simulink model "BuildingModelWithSolarLoad"  (R2024a)
settings: Solver=ode1be  StartTime=0.0  StopTime=522000  FixedStep=3600  MaxStep=3600  RelTol=1e-3  AbsTol=1e-3
PreLoadFcn:
  | % WallModelParams
libraries: fl_lib x12, nesl_utility x6
CloseFcn:
  | % clear flow out roomHeight wall win
settings Model: Creator=vikrants  LastModifiedBy=vikrants
settings SolverCC: AutoScaleAbsTol=off  AlgebraicLoopSolver=TrustRegion  MaxZcPerStep=1
settings DebuggingCC: UnconnectedInputMsg=warning  UnconnectedOutputMsg=warning  UnconnectedLineMsg=warning  SymbolicDimsDataTypeCodeGenerationDiagnostic=none
settings ModelReferenceCC: EnableRefExpFcnMdlSchedulingChecks=on
settings SFSimCC: CustomCodeUndefinedFunction=UseInterfaceOnly
settings RTWCC: GPUComputeCapability=3.5  DLArmComputeVersion=19.05
settings SimscapeCC: SimscapeLogType=all  SimscapeLogSimulationStatistics=on  SimscapeLogLimitData=off  SimscapeLogDataHistory=10000  SimscapeCompileComponentReuse=on  SimscapeMultithreadedCompilation=off

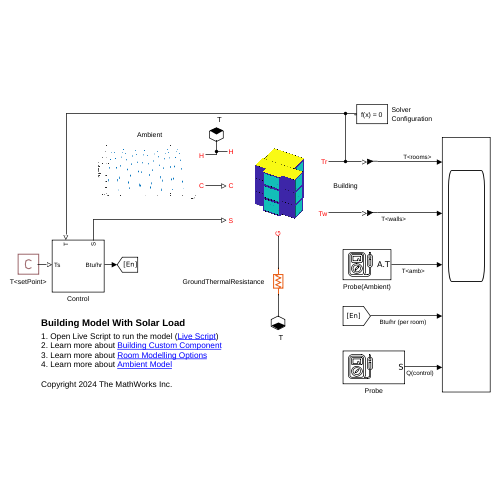
[thumbnail: Simulink's stored preview of the top-level diagram]
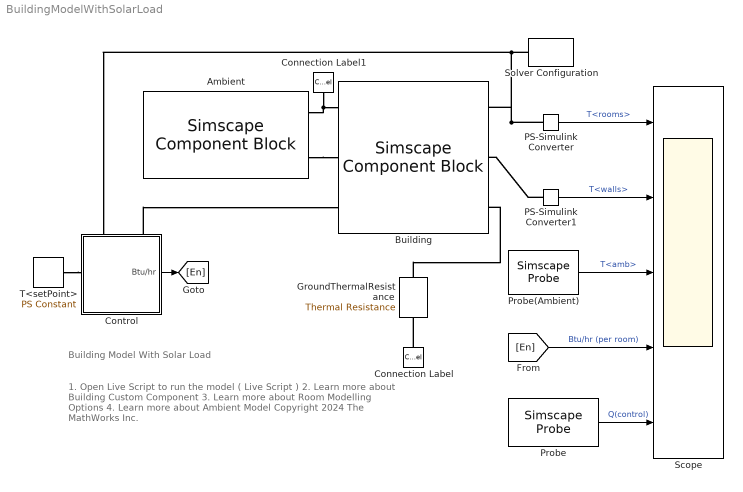
== system BuildingModelWithSolarLoad ==
  note: 1. Open Live Script to run the model ( Live Script )
      | 2. Learn more about Building Custom Component
      | 3. Learn more about Room Modelling Options
      | 4. Learn more about Ambient Model
      |
      | Copyright 2024 The MathWorks Inc.
  note: Building Model With Solar Load
  Ambient : SimscapeComponentBlock  SourceFile=EnvModel  ComponentPath=EnvModel  ComponentVariants="[\"EnvModel\"]"  ComponentVariantNames="[\"EnvModel\"]"  ClassName=EnvModel  SchemaVersion=1  listOfDays="[122  123  124  125  126  127  128] % Parameterized on :13-Nov-2024 08:59:39"  sunrise="[19381.846      19356.8068      19332.5383       19309.053      19286.3628      19264.4789      19243.4119] % Parameterized on :13-Nov-2024 08:59:39 s"  sunset="[67018.154      67043.1932      67067.4617       67090.947      67113.6372      67135.5211      67156.5881] % Parameterized on :13-Nov-2024 08:59:39 s"  startTime=3600 % Parameterized on :13-Nov-2024 08:59:39 s  avgDayTvec="[303  303  303  303  303  303  303] % Parameterized on :13-Nov-2024 08:59:39 K"  pcDayTvar=1 % Parameterized on :13-Nov-2024 08:59:39  avgNightTvec="[299  299  299  299  299  299  299] % Parameterized on :13-Nov-2024 08:59:39 K"  pcNightTvar=1 % Parameterized on :13-Nov-2024 08:59:39  cloudData=cloudCoverOptions.daily  cloudCoverVal="[0  0  0  0  0  0  0] % Parameterized on :13-Nov-2024 08:59:39"
      settings: CopyFcn=simscape.engine.sli.internal.componentblockcallback(gcbh,'COPY')  PreCopyFcn=simscape.engine.sli.internal.componentblockcallback(gcbh,'PRECOPY')  PreDeleteFcn=simscape.engine.sli.internal.componentblockcallback(gcbh,'PREDELETE')  InternalSimscapePortConfiguration="{\"Bottom\":[],\"Left\":[],\"Right\":[{\"id\":\"A\",\"label\":\"H\",\"type\":\"foundation.thermal.thermal\"},{\"id\":\"cloud\",\"label\":\"C\",\"type\":\"output\"}],\"Top\":[]}"
      mask Type: EnvModel
  Building : SimscapeComponentBlock  SourceFile=BuildingModel  ComponentPath=BuildingModel  ComponentVariants="[\"BuildingModel\"]"  ComponentVariantNames="[\"BuildingModel\"]"  ClassName=BuildingModel  SchemaVersion=1  nApts=3 % Parameterized on :13-Nov-2024 08:59:39  nRooms=4 % Parameterized on :13-Nov-2024 08:59:39  roomVolMat=[22.6534772736 39.6435852288 13.59208636416 9.9108963072;22.6534772736 39.6435852288 13.59208636416 9.9108963072;22.6534772736 39.6435852288 13.59208636416 9.9108963072] % Parameterized on :13-Nov-2024 08:59:39 m^3  roomConnMat=[1 1 1 2 1.9235928;1 1 1 3 7.1789544;1 1 1 4 6.2816232;1 2 1 3 0.48121824;1 2 1 4 0.9614916;2 1 2 2 1.9235928;2 1 2 3 7.1789544;2 1 2 4 6.2816232;2 2 2 3 0.48121824;2 2 2 4 0.9614916;3 1 3 2 1.9235928;3 1 3 3 7.1789544;3 1 3 4 6.2816232;3 2 3 3 0.48121824;3 2 3 4 0.9614916;1 1 2 1 7.4322432;1 2 2 2 13.0064256;1 3 2 3 4.45934592;1 4 2 4 3.2516064;2 1 3 1 7.4322432;2 2 3 2 13.0064256;2 3 3 3 4.45934592;2 4 3 4 3.2516064] % Parameterized on :13-Nov-2024 08:59:39  roomEnvConnMat=[1 1 1 2.22966 5.20254 0;1 1 2 2.536809318 0 0;1 1 4 3.094691833 0 0;1 2 2 9.2903 0 0;1 2 3 3.90192 9.10448 0;1 2 4 4.64515 4.64515 0;1 3 1 5.5742 0 0;1 3 3 1.165788188 0 0;1 3 4 2.22966 5.20254 0;1 4 1 4.6452 0 0;1 4 2 4.55224 1.95096 0;1 4 3 0.8698137 0 0;2 1 1 2.22966 5.20254 0;2 1 2 2.536809318 0 0;2 1 4 3.094691833 0 0;2 2 2 9.2903 0 0;2 2 3 3.90192 9.10448 0;2 2 4 4.64515 4.64515 0;2 3 1 5.5742 0 0;2 3 3 1.165788188 0 0;2 3 4 2.22966 5.20254 0;2 4 1 4.6452 0 0;2 4 2 4.55224 1.95096 0;2 4 3 0.8698137 0 0;3 1 1 2.22966 5.20254 0;3 1 2 2.536809318 0 0;3 1 4 3.094691833 0 0;3 2 2 9.2903 0 0;3 2 3 3.90192 9.10448 0;3 2 4 4.64515 4.64515 0;3 3 1 5.5742 0 0;3 3 3 1.165788188 0 0;3 3 4 2.22966 5.20254 0;3 4 1 4.6452 0 0;3 4 2 4.55224 1.95096 0;3 4 3 0.8698137 0 0] % Parameterized on :13-Nov-2024 08:59:39  roomEnvSolarRad=[0 0 0 0 0 0 0 0 0 0 0 0 508.7493 695.7679 740.5149 646.0261 443.1172 175.983 0 0 0 0 0 0 0 0 0 0 0 0 0 0 0 0 0 0 506.6863 693.3518 738.2975 644.5609 442.8175 177.0738 0 0 0 0 0 0 0 0 0 0 0 0 0 0 0 0 0 0 504.6328 690.9373 736.0614 643.0554 442.4581 178.0902 0 0 0 0 0 0 0 0 0 0 0 0 0 0 0 0 0 0 502.5917 688.5273 733.8098 641.5122 442.0409 179.033 0 0 0 0 0 0 0 0 0 0 0 0 0 0 0 0 0 0 500.5659 686.125 731.5459 639.9341 441.5678 179.9031 0 0 0 0 0 0 0 0 0 0 0 0 0 0 0 0 0 0 498.5584 683.7335 729.2727 638.3238 441.0408 180.7014 0 0 0 0 0 0 0;0 0 0 0 0 0 0 0 0 0 0 0 0 0 0 0 0 0 0 0 0 0 0 0 0 0 0 0 0 0 0 0 0 0 0 0 0 0 0 0 0 0 0 0 0 0 0 0 0 0 0 0 0 0 0 0 0 0 0 0 0 0 0 0 0 0 0 0 0 0 0 0 0 0 0 0 0 0 0 0 0 0 0 0 0 0 0 0 0 0 0 0 0 0 0 0 0 0 0 0 0 0 0 0 0 0 0 0 0 0 0 0 0 0 0 0 0 0 0 0 0 0 0 0 0 0 0 0 0 0 0 0 0 0 0 0 0 0 0 0 0 0 0 0 0;0 0 0 0 0 0 8.760353 103.49157 342.38462 691.35726 1034.3368 1231.5064 0 0 0 0 0 0 0 0 0 0 0 0 0 0 0 0 0 0 7.2840779 100.4301 337.93248 686.02689 1029.0281 1226.9589 1091.7999 0 0 0 0 0 0 0 0 0 0 0 0 0 0 0 0 0 5.8286813 97.427164 333.55914 680.76079 1023.7247 1222.29 1088.064 0 0 0 0 0 0 0 0 0 0 0 0 0 0 0 0 0 4.3944434 94.483934 329.26741 675.5639 1018.4336 1217.5127 1084.1895 0 0 0 0 0 0 0 0 0 0 0 0 0 0 0 0 0 2.98164 91.601534 325.05996 670.44102 1013.1618 1212.6398 1080.1838 0 0 0 0 0 0 0 0 0 0 0 0 0 0 0 0 0 1.5905448 88.78103 320.93937 665.39687 1007.9163 1207.6841 1076.055 0 0 0 0 0 0 0 0 0 0 0 0;0 0 0 0 0 0 0 0 0 0 0 0 0 0 0 0 0 0 0 0 0 0 0 0 0 0 0 0 0 0 0 0 0 0 0 0 0 0 0 0 0 0 0 0 0 0 0 0 0 0 0 0 0 0 0 0 0 0 0 0 0 0 0 0 0 0 0 0 0 0 0 0 0 0 0 0 0 0 0 0 0 0 0 0 0 0 0 0 0 0 0 0 0 0 0 0 0 0 0 0 0 0 0 0 0 0 0 0 0 0 0 0 0 0 0 0 0 0 0 0 0 0 0 0 0 0 0 0 0 0 0 0 0 0 0 0 0 0 0 0 0 0 0 0 0;0 0 0 0 0 0 0 0 0 0 0 0 0 0 0 0 0 0 0 0 0 0 0 0 0 0 0 0 0 0 0 0 0 0 0 0 0 0 0 0 0 0 0 0 0 0 0 0 0 0 0 0 0 0 0 0 0 0 0 0 0 0 0 0 0 0 0 0 0 0 0 0 0 0 0 0 0 0 0 0 0 0 0 0 0 0 0 0 0 0 0 0 0 0 0 0 0 0 0 0 0 0 0 0 0 0 0 0 0 0 0 0 0 0 0 0 0 0 0 0 0 0 0 0 0 0 0 0 0 0 0 0 0 0 0 0 0 0 0 0 0 0 0 0 0;0 0 0 0 0 0 8.760353 103.49157 342.38462 691.35726 1034.3368 1231.5064 0 0 0 0 0 0 0 0 0 0 0 0 0 0 0 0 0 0 7.2840779 100.4301 337.93248 686.02689 1029.0281 1226.9589 1091.7999 0 0 0 0 0 0 0 0 0 0 0 0 0 0 0 0 0 5.8286813 97.427164 333.55914 680.76079 1023.7247 1222.29 1088.064 0 0 0 0 0 0 0 0 0 0 0 0 0 0 0 0 0 4.3944434 94.483934 329.26741 675.5639 1018.4336 1217.5127 1084.1895 0 0 0 0 0 0 0 0 0 0 0 0 0 0 0 0 0 2.98164 91.601534 325.05996 670.44102 1013.1618 1212.6398 1080.1838 0 0 0 0 0 0 0 0 0 0 0 0 0 0 0 0 0 1.5905448 88.78103 320.93937 665.39687 1007.9163 1207.6841 1076.055 0 0 0 0 0 0 0 0 0 0 0 0;0 0 0 0 0 0 0 0 0 0 0 0 508.7493 695.7679 740.5149 646.0261 443.1172 175.983 0 0 0 0 0 0 0 0 0 0 0 0 0 0 0 0 0 0 506.6863 693.3518 738.2975 644.5609 442.8175 177.0738 0 0 0 0 0 0 0 0 0 0 0 0 0 0 0 0 0 0 504.6328 690.9373 736.0614 643.0554 442.4581 178.0902 0 0 0 0 0 0 0 0 0 0 0 0 0 0 0 0 0 0 502.5917 688.5273 733.8098 641.5122 442.0409 179.033 0 0 0 0 0 0 0 0 0 0 0 0 0 0 0 0 0 0 500.5659 686.125 731.5459 639.9341 441.5678 179.9031 0 0 0 0 0 0 0 0 0 0 0 0 0 0 0 0 0 0 498.5584 683.7335 729.2727 638.3238 441.0408 180.7014 0 0 0 0 0 0 0;0 0 0 0 0 0 0 0 0 0 0 0 0 0 0 0 0 0 0 0 0 0 0 0 0 0 0 0 0 0 0 0 0 0 0 0 0 0 0 0 0 0 0 0 0 0 0 0 0 0 0 0 0 0 0 0 0 0 0 0 0 0 0 0 0 0 0 0 0 0 0 0 0 0 0 0 0 0 0 0 0 0 0 0 0 0 0 0 0 0 0 0 0 0 0 0 0 0 0 0 0 0 0 0 0 0 0 0 0 0 0 0 0 0 0 0 0 0 0 0 0 0 0 0 0 0 0 0 0 0 0 0 0 0 0 0 0 0 0 0 0 0 0 0 0;0 0 0 0 0 0 8.760353 103.49157 342.38462 691.35726 1034.3368 1231.5064 0 0 0 0 0 0 0 0 0 0 0 0 0 0 0 0 0 0 7.2840779 100.4301 337.93248 686.02689 1029.0281 1226.9589 1091.7999 0 0 0 0 0 0 0 0 0 0 0 0 0 0 0 0 0 5.8286813 97.427164 333.55914 680.76079 1023.7247 1222.29 1088.064 0 0 0 0 0 0 0 0 0 0 0 0 0 0 0 0 0 4.3944434 94.483934 329.26741 675.5639 1018.4336 1217.5127 1084.1895 0 0 0 0 0 0 0 0 0 0 0 0 0 0 0 0 0 2.98164 91.601534 325.05996 670.44102 1013.1618 1212.6398 1080.1838 0 0 0 0 0 0 0 0 0 0 0 0 0 0 0 0 0 1.5905448 88.78103 320.93937 ...(+11544 chars)] % Parameterized on :13-Nov-2024 08:59:39  floorGroundConn=[1 1 7.4322432;1 2 13.0064256;1 3 4.45934592;1 4 3.2516064] % Parameterized on :13-Nov-2024 08:59:39  roomModelOption=roomPhysicsOptions.requirements  roomRadiatorArea=ones(5, 8) m^2  roomUFPipingArea=ones(5, 8) m^2  roofEnvConnMat=[3 1 7.4322432;3 2 13.0064256;3 3 4.45934592;3 4 3.2516064] % Parameterized on :13-Nov-2024 08:59:39  roofEnvSolarRad=[0 0 0 0 0 0 59.37688 284.0187 558.4148 731.6277 703.3205 481.3691 548.3154 730.7268 705.3155 494.6307 218.2659 27.22395 0 0 0 0 0 0 0 0 0 0 0 0 59.62248 284.8127 560.2036 735.0546 709.0017 490.7252 555.3351 735.4838 708.7842 497.1489 219.8792 27.78296 0 0 0 0 0 0 0 0 0 0 0 0 59.88223 285.6142 561.9659 738.4099 714.5914 500.0937 562.4302 740.1887 712.1618 499.5757 221.4311 28.32576 0 0 0 0 0 0 0 0 0 0 0 0 60.15639 286.4239 563.703 741.6939 720.0859 509.4443 569.5843 744.8379 715.4469 501.9099 222.9203 28.85136 0 0 0 0 0 0 0 0 0 0 0 0 60.44522 287.2427 565.4158 744.9067 725.4816 518.7498 576.781 749.4277 718.6383 504.1509 224.3458 29.3588 0 0 0 0 0 0 0 0 0 0 0 0 60.74897 288.0714 567.1056 748.0487 730.7754 527.9854 584.0035 753.9547 721.7348 506.2978 225.7066 29.84717 0 0 0 0 0 0 0;0 0 0 0 0 0 59.37688 284.0187 558.4148 731.6277 703.3205 481.3691 548.3154 730.7268 705.3155 494.6307 218.2659 27.22395 0 0 0 0 0 0 0 0 0 0 0 0 59.62248 284.8127 560.2036 735.0546 709.0017 490.7252 555.3351 735.4838 708.7842 497.1489 219.8792 27.78296 0 0 0 0 0 0 0 0 0 0 0 0 59.88223 285.6142 561.9659 738.4099 714.5914 500.0937 562.4302 740.1887 712.1618 499.5757 221.4311 28.32576 0 0 0 0 0 0 0 0 0 0 0 0 60.15639 286.4239 563.703 741.6939 720.0859 509.4443 569.5843 744.8379 715.4469 501.9099 222.9203 28.85136 0 0 0 0 0 0 0 0 0 0 0 0 60.44522 287.2427 565.4158 744.9067 725.4816 518.7498 576.781 749.4277 718.6383 504.1509 224.3458 29.3588 0 0 0 0 0 0 0 0 0 0 0 0 60.74897 288.0714 567.1056 748.0487 730.7754 527.9854 584.0035 753.9547 721.7348 506.2978 225.7066 29.84717 0 0 0 0 0 0 0;0 0 0 0 0 0 59.37688 284.0187 558.4148 731.6277 703.3205 481.3691 548.3154 730.7268 705.3155 494.6307 218.2659 27.22395 0 0 0 0 0 0 0 0 0 0 0 0 59.62248 284.8127 560.2036 735.0546 709.0017 490.7252 555.3351 735.4838 708.7842 497.1489 219.8792 27.78296 0 0 0 0 0 0 0 0 0 0 0 0 59.88223 285.6142 561.9659 738.4099 714.5914 500.0937 562.4302 740.1887 712.1618 499.5757 221.4311 28.32576 0 0 0 0 0 0 0 0 0 0 0 0 60.15639 286.4239 563.703 741.6939 720.0859 509.4443 569.5843 744.8379 715.4469 501.9099 222.9203 28.85136 0 0 0 0 0 0 0 0 0 0 0 0 60.44522 287.2427 565.4158 744.9067 725.4816 518.7498 576.781 749.4277 718.6383 504.1509 224.3458 29.3588 0 0 0 0 0 0 0 0 0 0 0 0 60.74897 288.0714 567.1056 748.0487 730.7754 527.9854 584.0035 753.9547 721.7348 506.2978 225.7066 29.84717 0 0 0 0 0 0 0;0 0 0 0 0 0 59.37688 284.0187 558.4148 731.6277 703.3205 481.3691 548.3154 730.7268 705.3155 494.6307 218.2659 27.22395 0 0 0 0 0 0 0 0 0 0 0 0 59.62248 284.8127 560.2036 735.0546 709.0017 490.7252 555.3351 735.4838 708.7842 497.1489 219.8792 27.78296 0 0 0 0 0 0 0 0 0 0 0 0 59.88223 285.6142 561.9659 738.4099 714.5914 500.0937 562.4302 740.1887 712.1618 499.5757 221.4311 28.32576 0 0 0 0 0 0 0 0 0 0 0 0 60.15639 286.4239 563.703 741.6939 720.0859 509.4443 569.5843 744.8379 715.4469 501.9099 222.9203 28.85136 0 0 0 0 0 0 0 0 0 0 0 0 60.44522 287.2427 565.4158 744.9067 725.4816 518.7498 576.781 749.4277 718.6383 504.1509 224.3458 29.3588 0 0 0 0 0 0 0 0 0 0 0 0 60.74897 288.0714 567.1056 748.0487 730.7754 527.9854 584.0035 753.9547 721.7348 506.2978 225.7066 29.84717 0 0 0 0 0 0 0] % Parameterized on :13-Nov-2024 08:59:39  radiatorPipeGap=1e-2 m  radiatorPipeHydrDia=5e-3 m  radiatorPipeArea=2e-5 m^2  UFPipeGap=1e-1 m  UFPipeHydrDia=5e-3 m  UFPipeArea=2e-5 m^2  wallAbsorptivity=.6  wallThickness=0.3 m  wallMaterialDen=2400 kg/m^3  wallMaterialCp=1500 J/(K*kg)  wallThermalK=2.25 W/(K*m)  winAbsorptivity=.4  winTransmissivity=.2  winThickness=.01 m  winMaterialDen=4000 kg/m^3  winMaterialCp=840 J/(K*kg)  winThermalK=1 W/(K*m)  heatTransferPipeRoughness=1e-06 m  extToWallHTC=5 W/(K*m^2)  intToRoomHTC=5 W/(K*m^2)  iniTemperature=299 % Parameterized on :13-Nov-2024 08:59:39 K  airDensity=1.28 kg/m^3  airCp=700 J/(K*kg)  minArea=1e-10 m^2
      settings: CopyFcn=simscape.engine.sli.internal.componentblockcallback(gcbh,'COPY')  PreCopyFcn=simscape.engine.sli.internal.componentblockcallback(gcbh,'PRECOPY')  PreDeleteFcn=simscape.engine.sli.internal.componentblockcallback(gcbh,'PREDELETE')  InternalSimscapePortConfiguration="{\"Bottom\":[{\"id\":\"G\",\"label\":\"G\",\"type\":\"foundation.thermal.thermal\"}],\"Left\":[{\"id\":\"H\",\"label\":\"H\",\"type\":\"foundation.thermal.thermal\"},{\"id\":\"C\",\"label\":\"C\",\"type\":\"input\"},{\"id\":\"S\",\"label\":\"S\",\"type\":\"input\"}],\"Right\":[{\"id\":\"roomTemp\",\"label\":\"Tr\",\"type\":\"output\"},{\"id\":\"wallTemp\",\"label\":\"Tw\",\"type\":\"output\"}],\"Top\":[]}"
      mask Type: BuildingModel
  Connection Label : ConnectionLabel  Label=T
  Connection Label1 : ConnectionLabel  Label=T
  Control : Subsystem
      settings: PortSchema="{\"entries\":[{\"content\":{\"sides\":[{\"content\":{\"connectorIds\":[\"Out1\"]},\"type\":\"ConnectorPlacement.EquallySpacedRectSide\",\"uuid\":\"bf0d3f6c-4199-48ed-9d1b-942d678a196d\"},{\"content\":{\"connectorIds\":[\"RConn1\"],\"side\":\"RIGHT\"},\"type\":\"ConnectorPlacement.EquallySpacedRectSide\",\"uuid\":\"048b5b2b-ccfc-4083-80b1-51c1896923e2\"},{\"content\":{\"side\":\"TOP\"},\"type\":\"ConnectorPlacement.EquallySpacedRectSide\",\"uuid\":\"550f74ea-2758-4466-8134-2f10276d8ab6\"},{\"content\":{\"connectorIds\":[\"RConn2\",\"RConn3\"],\"side\":\"BOTTOM\"},\"type\":\"ConnectorPlacement.EquallySpacedRectSide\",\"uuid\":\"b8e21315-4710-4fb3-a2ab-c08e79356caa\"}]},\"type\":\"ConnectorPlacement.EquallySpacedConnector\",\"uuid\":\"91aadc23-894a-4dd0-ab72-650090e5f490\"}],\"packageUris\":[\"http://schema.mathworks.com/mf0/Connector/R2020b\"],\"version\":\"1.0\"}"
  GroundThermalResistance : fl_lib/Thermal/Thermal Elements/Thermal Resistance  resistance=100 % Parameterized on :13-Nov-2024 08:59:39 K/W  T_specify=off  T_priority=None  T=0 K  T_nominal_specify=off  T_nominal_value=1  T_nominal_unit=K  Q_specify=off  Q_priority=None  Q=0 W  Q_nominal_specify=off  Q_nominal_value=1  Q_nominal_unit=W
  PS-Simulink Converter : nesl_utility/PS-Simulink Converter  PhysicalDomain=network_engine_domain  SubClassName=ps_output  LeftPortType=input  RightPortType=output  PseudoPeriodic=off  Frequencies=[]  VectorFormat=inherit  Unit=inherit  AffineConversion=off
  PS-Simulink Converter1 : nesl_utility/PS-Simulink Converter  PhysicalDomain=network_engine_domain  SubClassName=ps_output  LeftPortType=input  RightPortType=output  PseudoPeriodic=off  Frequencies=[]  VectorFormat=inherit  Unit=inherit  AffineConversion=off
  Probe : SimscapeProbe  BoundBlock=49  Variables={S}
  Probe(Ambient) : SimscapeProbe  BoundBlock=267  Variables={A.T}
  Scope : Scope  NumInputPorts=5
  Solver Configuration : nesl_utility/Solver Configuration  PhysicalDomain=network_engine_domain  SubClassName=solver  LeftPortType=input  RightPortType=generic  Tones=[]  Harmonics=[]  SimulateNoise=off  Profile=off  UseLocalSampling=off  EnableSwitchedLinearOptims=on  FrequencyDomain=off  UseCCode=off  RelTol=0.001  AbsTol=1e-06  MinStep=1e-09  ToWorkspace=off  RevertToSquareIcSolve=off  NumHomotopyIterations=100  PhasorMode=off  PhasorModeNumHarmonics=1  ConsistencySolver=NEWTON_XTOL_AFTER_FTOL  IndexReductionMethod=DerivativeReplacement  DoDC=off  ResidualTolerance=1e-09  ConsistencyTolSource=GLOBAL  ConsistencyAbsTol=0.001  ConsistencyRelTol=0.001  ConsistencyTolFactor=0.001  UseLocalSolver=off  LocalSolverChoice=NE_BACKWARD_EULER_ADVANCER  ResolveIndetEquations=on  FunctionEvalNumThread=1  LocalSolverSampleTime=3600  DoFixedCost=off  MaxNonlinIter=3  MaxModeIter=2  ComputeImpulses=off  ImpulseIterations=2  LinearAlgebra=auto  LinearAlgebraNumThread=0  EquationFormulation=NE_TIME_EF  DelaysMemoryBudget=1024  AutomaticFiltering=on  FilteringTimeConstant=0.001  PartitionStorageMethod=AS_NEEDED  PartitionMemoryBudget=1024  PartitionMethod=ROBUST  MultibodyUseLocalSolver=off  MultibodyLocalSolverChoice=ODE1  MultibodyLocalSolverSampleTime=0.001
  T<setPoint> : fl_lib/Physical Signals/Sources/PS Constant  constant=293 % Parameterized on :13-Nov-2024 08:59:39 K
  wires:
  Probe(Ambient)/1 -> Scope/3  "T<amb>"
  PS-Simulink Converter/1 -> Scope/1  "T<rooms>"
  PS-Simulink Converter1/1 -> Scope/2  "T<walls>"
  Control/1(Btu/hr) -> [En]
  [En] -> Scope/4  "Btu/hr (per room)"
  Probe/1 -> Scope/5  "Q(control)"
  connections:
  PS-Simulink Converter1/LConn1 -- Building/RConn2
  Ambient/RConn1 -- Connection Label1/LConn1 -- Building/LConn1
  PS-Simulink Converter/LConn1 -- Solver Configuration/RConn1 -- Control/RConn3 -- Building/RConn1
  Control/RConn2 -- Building/LConn3
  T<setPoint>/RConn1 -- Control/RConn1
  Ambient/RConn2 -- Building/LConn2
  Connection Label/LConn1 -- GroundThermalResistance/RConn1
  GroundThermalResistance/LConn1 -- Building/RConn3

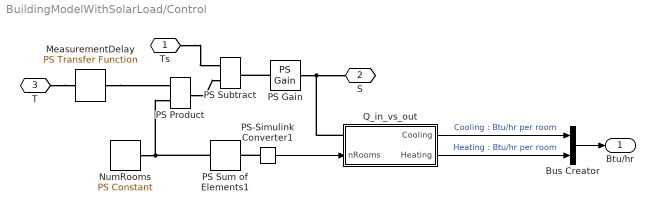
== system BuildingModelWithSolarLoad/Control ==
  Bus Creator : BusCreator  Inputs=2
  MeasurementDelay : fl_lib/Physical Signals/Linear Operators/PS Transfer Function  transfer_function_type=foundation.enum.transfer_function_type.lag  T=1 s  T1=2 s  T2=1 s  reset_method=foundation.enum.IntegratorResetSpec.None  initial_condition_spec=foundation.enum.IntegratorICSpec.Internal  y0=299 % Parameterized on :13-Nov-2024 08:59:39 K
      settings: InternalSimscapePortConfiguration="{\"Bottom\":[],\"Left\":[{\"id\":\"U\",\"label\":\"\",\"type\":\"input\"}],\"Right\":[{\"id\":\"Y\",\"label\":\"\",\"type\":\"output\"}],\"Top\":[]}"
  NumRooms : fl_lib/Physical Signals/Sources/PS Constant  constant=[[1 1 1 1;1 1 1 1;1 1 1 1]] % Parameterized on :13-Nov-2024 08:59:39
  PS Gain : fl_lib/Physical Signals/Functions/PS Gain  gain=200000 W/K
  PS Product : fl_lib/Physical Signals/Functions/PS Product
  PS Subtract : fl_lib/Physical Signals/Functions/PS Subtract
  PS Sum of Elements1 : fl_lib/Physical Signals/Functions/PS Sum of Elements  sumAll=true
      settings: InternalSimscapePortConfiguration="{\"Bottom\":[],\"Left\":[{\"id\":\"I\",\"label\":\"\",\"type\":\"input\"}],\"Right\":[{\"id\":\"O\",\"label\":\"\",\"type\":\"output\"}],\"Top\":[]}"
  PS-Simulink Converter1 : nesl_utility/PS-Simulink Converter  PhysicalDomain=network_engine_domain  SubClassName=ps_output  LeftPortType=input  RightPortType=output  PseudoPeriodic=off  Frequencies=[]  VectorFormat=inherit  Unit=inherit  AffineConversion=off
  Q_in_vs_out : Subsystem
      settings: PortSchema="{\"entries\":[{\"content\":{\"sides\":[{\"content\":{\"connectorIds\":[\"LConn1\",\"In1\"]},\"type\":\"ConnectorPlacement.EquallySpacedRectSide\",\"uuid\":\"1772fb37-9fba-4a8a-b11f-78a26f95d83b\"},{\"content\":{\"connectorIds\":[\"Out1\",\"Out2\"],\"side\":\"RIGHT\"},\"type\":\"ConnectorPlacement.EquallySpacedRectSide\",\"uuid\":\"e1c188bc-b6f5-4ee9-bf64-bac0a6ddf807\"},{\"content\":{\"side\":\"TOP\"},\"type\":\"ConnectorPlacement.EquallySpacedRectSide\",\"uuid\":\"71c9bd2e-a995-40c2-93b9-42b8904a6810\"}]},\"type\":\"ConnectorPlacement.EquallySpacedConnector\",\"uuid\":\"7220c813-1faf-443a-9d27-ed3416786eaf\"}],\"packageUris\":[\"http://schema.mathworks.com/mf0/Connector/R2020b\"],\"version\":\"1.0\"}"
  Ts : PMIOPort  Side=Right
  S : PMIOPort  Port=2  Side=Right
  T : PMIOPort  Port=3  Side=Right
  Btu/hr : Outport
  wires:
  Q_in_vs_out/1(Cooling) -> Bus Creator/1  "Cooling : Btu/hr per room"
  Q_in_vs_out/2(Heating) -> Bus Creator/2  "Heating : Btu/hr per room"
  Bus Creator/1 -> Btu/hr/1
  PS-Simulink Converter1/1 -> Q_in_vs_out/1(nRooms)
  connections:
  Ts/RConn1 -- PS Subtract/LConn1
  PS Product/RConn1 -- PS Subtract/LConn2
  MeasurementDelay/RConn1 -- PS Product/LConn1
  NumRooms/RConn1 -- PS Product/LConn2 -- PS Sum of Elements1/LConn1
  PS-Simulink Converter1/LConn1 -- PS Sum of Elements1/RConn1
  PS Gain/LConn1 -- PS Subtract/RConn1
  PS Gain/RConn1 -- Q_in_vs_out/LConn1 -- S/RConn1
  T/RConn1 -- MeasurementDelay/LConn1

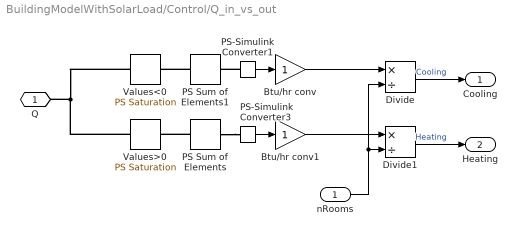
== system BuildingModelWithSolarLoad/Control/Q_in_vs_out ==
  nRooms : Inport
  Btu/hr conv : Gain
  Btu/hr conv1 : Gain
  Divide : Product  Inputs=*/
  Divide1 : Product  Inputs=*/
  PS Sum of Elements : fl_lib/Physical Signals/Functions/PS Sum of Elements  sumAll=true
      settings: InternalSimscapePortConfiguration="{\"Bottom\":[],\"Left\":[{\"id\":\"I\",\"label\":\"\",\"type\":\"input\"}],\"Right\":[{\"id\":\"O\",\"label\":\"\",\"type\":\"output\"}],\"Top\":[]}"
  PS Sum of Elements1 : fl_lib/Physical Signals/Functions/PS Sum of Elements  sumAll=true
      settings: InternalSimscapePortConfiguration="{\"Bottom\":[],\"Left\":[{\"id\":\"I\",\"label\":\"\",\"type\":\"input\"}],\"Right\":[{\"id\":\"O\",\"label\":\"\",\"type\":\"output\"}],\"Top\":[]}"
  PS-Simulink Converter1 : nesl_utility/PS-Simulink Converter  PhysicalDomain=network_engine_domain  SubClassName=ps_output  LeftPortType=input  RightPortType=output  PseudoPeriodic=off  Frequencies=[]  VectorFormat=inherit  Unit=inherit  AffineConversion=off
  PS-Simulink Converter3 : nesl_utility/PS-Simulink Converter  PhysicalDomain=network_engine_domain  SubClassName=ps_output  LeftPortType=input  RightPortType=output  PseudoPeriodic=off  Frequencies=[]  VectorFormat=inherit  Unit=inherit  AffineConversion=off
  Values<0 : fl_lib/Physical Signals/Nonlinear Operators/PS Saturation  upper_limit=0 J/s  lower_limit=-inf J/s
  Values>0 : fl_lib/Physical Signals/Nonlinear Operators/PS Saturation  upper_limit=inf J/s  lower_limit=0 J/s
  Q : PMIOPort  Side=Left
  Cooling : Outport
  Heating : Outport  Port=2
  wires:
  PS-Simulink Converter3/1 -> Btu/hr conv1/1
  PS-Simulink Converter1/1 -> Btu/hr conv/1
  Btu/hr conv1/1 -> Divide1/1
  Divide1/1 -> Heating/1  "Heating"
  nRooms/1 -> Divide/2, Divide1/2
  Divide/1 -> Cooling/1  "Cooling"
  Btu/hr conv/1 -> Divide/1
  connections:
  PS Sum of Elements1/LConn1 -- Values<0/RConn1
  PS Sum of Elements/LConn1 -- Values>0/RConn1
  PS-Simulink Converter1/LConn1 -- PS Sum of Elements1/RConn1
  Values>0/LConn1 -- Values<0/LConn1 -- Q/RConn1
  PS Sum of Elements/RConn1 -- PS-Simulink Converter3/LConn1
